simulink library "rov_design_analysis"  (Simulink 6.0)
settings: Solver=ode45  SolverMode=SingleTasking  StartTime=0.0  StopTime=10.0  RelTol=1e-3
undefined symbols (not defined in the file or in its folder): amp, At, B, Bt, Ct, cycles, D, den, DL, Do, DQ, DQL, freq, frtest, I, L, m, M, Ma, magnitude, MaU, Mt, nmiss, num, phase, rg, sigbuilder_block, slcm, T, W, xb, xg, Xudot, yb, yg, Yvdot, zb, zg, Zwdot
libraries: simulink_extras x32, simulink x27, rov_design_analysis x15, marine_gnc x10, dspmtrx2 x6, dspstat3 x4
(part 1 of 9)
Description:
  | jkgkh
settings Model: LastModifiedBy=c chin
settings OptimizationCC: BooleanDataType=off
settings DebuggingCC: SolverPrmCheckMsg=none
settings HardwareCC: TargetUnknown=on

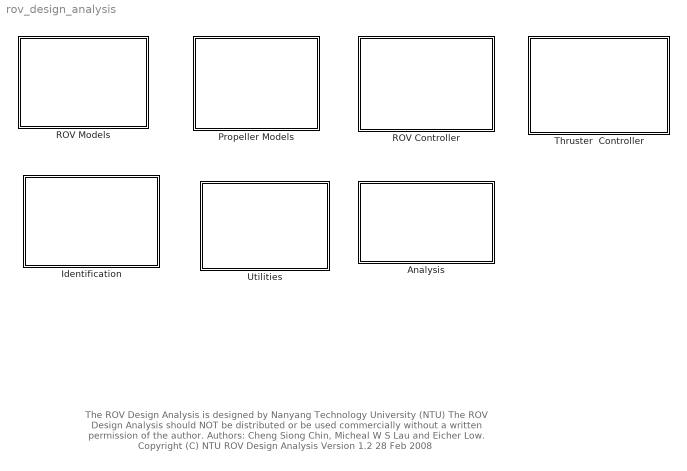
== system rov_design_analysis ==
  note: The ROV Design Analysis is designed by
      |
      |   Nanyang Technology University (NTU)
      |
      |
      | The ROV Design Analysis should NOT be distributed or be
      | used commercially without a written permission of the author.
      |
      |
      | Authors: Cheng Siong Chin, Micheal W S Lau
      | and  Eicher Low.
      |  Copyright (C)  NTU
      |
      |  ROV Design Analysis Version 1.2
      |  28 Feb 2008
  Analysis : Subsystem  AncestorBlock=rov_design_analysis/Scope
  Identification : Subsystem  AncestorBlock=rov_design_analysis/Scope
  Propeller Models : Subsystem  AncestorBlock="marine_gnc/Control/Dynamic  Positioning"
  ROV Models : Subsystem  AncestorBlock=marine_gnc/Control/Autopilots
  "ROV Controller " : Subsystem
  Thruster  Controller : Subsystem  AncestorBlock=|
      | rov_design_analysis/ROV Controller
      | Design
      | Applications
  Utilities : Subsystem  AncestorBlock=rov_design_analysis/ROV Modelling

== system rov_design_analysis/Analysis ==
  Linear/Nonlinear ROV Analysis : Subsystem  AncestorBlock=rov_design_analysis/Analysis/9. Design scaling
      settings: OpenFcn=|
      | clc
      | 
      | cd c:\Matlab7\toolbox\rov_design_analysis\gui
      | rov_property2
      mask Display: disp('ROV Property Analysis')
  Model Info : Subsystem  AncestorBlock=|  LoadFcn=slcm LoadBlock;  InitFcn=slcm('UpdateAllCMBlocksInThisModelInit')  mask(CMBlock){InitialSaveTempField=, InitialBlockCM=None, BlockCM=None, Frame=on, SaveTempField=, DisplayStringWithTags=|, MaskDisplayString=Reference:\n\nC. S. Chin, M. W. S. Lau, E. Low, G. G. Seet.\n Software for Modelling and Simulation of a Remotely Operated Vehicle, International Journal\nof Simulation Modelling, Vol.5, No. 3, p114-125, Sept 2006.\n\nAuthor: C.S.Chin\n27-Mar-2008 08:24:59, HorizontalTextAlignment=Left, LeftAlignmentValue=0.02, SourceBlockDiagram=rov_design_analysis, TagMaxNumber=20, CMTag1=, CMTag2=, CMTag3=, CMTag4=, CMTag5=, CMTag6=, CMTag7=, CMTag8=, CMTag9=, CMTag10=, CMTag11=, CMTag12=, CMTag13=, CMTag14=, CMTag15=, CMTag16=, CMTag17=, CMTag18=, CMTag19=, CMTag20=}
      | rov_design_analysis/ROV
      | Models/1. Nonlinear RRC ROV- unperturbed
      | (6DoF)/Model Info
      mask DisplayStringWithTags=|
      | Reference:\n
      | C. S. Chin, M. W. S. Lau, E. Low, G. G. Seet.\n Software for Modelling and Simulation of a Remotely Operated Vehicle, International Journal
      | of Simulation Modelling, Vol.5, No. 3, p114-125, Sept 2006.\n
      | %<Creator>Author: C.S.Chin
      | %<LastModificationDate>
      mask help: This block allows revision control information to be displayed within the model.
      settings: CopyFcn=slcm CopyBlock;  DeleteFcn=slcm Cancel;  PostSaveFcn=slcm('UpdateAllCMBlocksInThisModel')  NameChangeFcn=slcm Rename;  OpenFcn=slcm
      mask Display: text(str2num(LeftAlignmentValue), 0.5, MaskDisplayString, 'HorizontalAlignment', HorizontalTextAlignment)

== system rov_design_analysis/Identification ==
  Frequency Response Analysis : Subsystem
      mask Display: disp('Frequency Response \n Analysis')
  "Kalman filter  " : Subsystem  AncestorBlock=marine_gnc/Navigation/Observers/Kalman filter based autopilot wave filter  mask{lambda=0.1, w_o=1.0, T_b=1000, K=0.1, T=100, r=1, q1=100, q2=0.01, q3=0.01, P0=1*eye(5)}
      mask prompts: lambda "Relative damping ratio of wave spectrum: lambda"; w_o "Peak frequency of wave spectrum: w_o (rad/s)"; T_b "Bias time constant: T_b (s)"; K "Nomoto gain constant: K (1/s)"; T "Nomoto time constant: T (s)"; r "Compass variance: r"; q1 "Wave model variance: q1"; q2 "Ship model variance: q2"; q3 "Bias model variance: q3"; P0 "Initial covariance matrix"
      mask help:
      | Copyright (C) 2006 NTU
      | Author:  C.S.Chin
      mask Display: disp('Kalman filter')
  kalman filter- observer + i/o noise : Subsystem
      mask Display: disp('Kalman Filter')

== system rov_design_analysis/Propeller Models ==
  1.  propeller with motor characteristics - 1DoF (account for dynamic variation in ua,up) : Subsystem
      mask Type: Open-water propeller characteristics
      mask Description:
      | 1> Calculate the thrust and torque of a fixed pitch propeller, based on a polynomial representation of thrust and torque coefficients Kt and Kq from the open-water
      | characteristics. Kt and Kq are defined as polynomials alpha and beta in the advance number J=ua/(nD):
      | Kt =alpha(1)*J + alpha(2)
      | Kq =beta(1)*J + beta(2)
      | where n is the shaft speed, D the propeller diameter and ua the advance velocity of the propeller. The relationship between the thrust Ta and torque Qa are:
      | 
      | Ta = p*D^4*alpha(2)*n*|n| - p*D^3*alpha(1)*ua/(1+aT)
      | Qa = p*D^5*beta(2)*n*|n| - p*D^4*beta(1)*ua /(1+aQ)
      | where p is the density of water , n is the rotational speed of the propeller, aQ and aT are the constant used to account for dynamic variation in axial water speed.
      | 
      | 2> Calculate the Electrical DC Motor shaft equation:
      | Jdot*ndot+Km*Ke*n/Rm=Km*Vm/Rm-Qa
      | where Jm, Km, Ke, Rm are the motor constant and Vm is the voltage input.
      | 
      | 3>Calculate the axial flow velocity, up of the propeller
      | mt*updot-dto*up+dt|up|(up-ua)=Ta
      | where mt=gamma*p*Ap*l, gamma is an empirically determined added
      | mass coefficent, dt=2*p*Ap and advance velocity of propeller
      | 
      | ua=(1-W)u.
      | where W>0 is the wake fraction number (typical 0.1-0.4) and u is the ROV surge velocity.
      | 
      | *Note that ua is the advance velocity at the upstream of the propeller while up is axial
      |  velocity at the propeller. Details of the derivation can be found in:
      | 
      | [1] T.I.Fossen, M Blanke, Nonlinear output feedback control of underwater vehicle
      | propellers feedback form estimated axial flow velocity, IEEE Journal of Oceanic
      | Engineering, Vol 25, No.2, 2000.
      | 
      | Copyright (C) 2006 NTU, Author: C.S.Chin
      mask Display:
      | port_label('input', 1, 'volt [v]')
      | port_label('input', 2, 'vel [m/s & rad/s]')
      | port_label('output', 1, 'Ta [N]')
      | port_label('output', 2, 'Qa [Nm]')
      | port_label('output',3, 'ua[m/s]')
  2. propeller with motor characteristics - 1DoF (account for ua only) : Subsystem  AncestorBlock=|
      | rov_design_analysis/Propeller
      | Models/6. propeller with motor
      | characteristics
      | (account for ua)
      mask Type: Open-water propeller characteristics
      mask Description:
      | 1> Calculate the thrust and torque of a fixed pitch propeller, based on a polynomial representation of thrust and torque coefficients Kt and Kq from the open-water
      | characteristics. Kt and Kq for both thrust and torque are defined as:
      | 
      | Ktdo =p*Ap*l / (40*Kr) ,  Ktd=p*Ap/(800*Kr^2)         (Forward)
      | Ktdo = -p*Ap*l/(54Kr)  , Ktd=-p*Ap/(1458*Kr^2)       (Reverse)
      | 
      | Kqdo=p*Ap*l*D/(40*Kr) , Kqd=p*Ap*D/(800*Kr^2)     (Forward)
      | Kqdo=-p*Ap*l*D/(54*Kr), Kqd=-p*Ap*D/(1458*Kr^2)  (Reverse)
      | 
      | where p is the density of seawater=1024kg/m^3, l is the characteristic length =0.1m
      | Ap the propeller cross-sectional area, D is the propeller diameter =0.1m,
      | Kr=1.923, and  ua is the advance velocity of the propeller.
      | 
      | ua=(1-W)u
      | 
      | where W> 0 (=0.4) is the wake fraction number and u is the ROV surge velocity.
      | 
      | The relationship between the thrust Ta and torque Qa are:
      | 
      | Ta= Ktdo * ndot+Ktd*n|n|
      | Qa =Kqdo*ndot+Kqt*n|n|
      | where  n is the rotational speed of the propeller,
      | Ktdo=0.0104 ,Ktd=0.0027, Kqdo=0.00104, Kqd=0.00149.
      | 
      | 2> Calculate the Electrical DC Motor shaft equation:
      | Jdot*ndot+Kv*n=Km*Vm/Rm-Qa
      | where Jm = shaft inertia,
      |             Rm = motor resistance,
      |              Kv  = viscous friction coefficient,
      |             Vm = voltage input
      |             Qa =  torque output.
      | 
      | Copyright (C) 2006 NTU, Author: C.S.Chin
      mask Display:
      | port_label('input', 1, 'volt [v]')
      | port_label('input', 2, 'vel [m/s & rad/s]')
      | port_label('output', 1, 'Ta [N]')
      | port_label('output', 2, 'Qa [Nm]')
      | port_label('output',3, 'ua[m/s]')
  3. propeller with motor characteristics - 1DoF (no account for ua,up) : Subsystem
      mask Type: Propeller dynamic without considering axial velocity
      mask Description:
      | 1> Voltage input to motor:
      | 
      | Vm=Rm*I+Ke*Ohm+Lm*dI/dt
      | 
      | where Rm= motor resistance in Ohms
      |              Ke = motor  back emf constant in Vs/rad
      |              Lm= motor inductance in H
      |              I = motor current in A
      | 
      |  2> Propeller thrust (T) and torque (Q) output
      | 
      | T=Ktd*n|n|+Ktdo*n
      | Q=Kqd*n|n|+Kqdo*n
      | 
      | where n= rotational speed in rad/s
      | 
      | Copyright (C) 2006 NTU
      | Author:  C.S.Chin
  4. Open-water propeller characteristics : Subsystem  AncestorBlock=marine_gnc/Models/Propulsion/Open-water propeller characteristics  mask(Open-water propeller characteristics){Par_Thruster_D=1, Par_Thruster_Ktp=[-0.1060 -0.3246 0.4594], Par_Thruster_Kqp=[-0.0186 -0.0399 0.0680], Par_Thruster_reverse_reduction=0.8, Glob_rhow=1025}
      mask prompts: Par_Thruster_D "Thruster diameter [m]"; Par_Thruster_Ktp "Kt polynomial Ktp"; Par_Thruster_Kqp "Kq polynomial Kqp"; Par_Thruster_reverse_reduction "Reverse direction thrust reduction factor [-]"; Glob_rhow "Density of seawater [kg/m^3]"
      mask help:
      | Calculate the thrust and torque of a fixed pitch propeller, based on a polynomial representation of thrust and torque coefficients Kt and Kq from the open-water characteristics. Kt and Kq are defined as polynomials Ktp and Kqp in the advance number J=Va/(nD):
      |
      | Kt = Ktp(1)*J^2 + Kqp(2)*J + Kqp(3)
      | Kq = Kqp(1)*J^2 + Kqp(2)*J + Kqp(3)
      |
      | where n is the shaft speed, D the propelelr diameter and Va the advance velocity of the propeller. The relationship between the thrust T and torque Q and the coefficients Kt and Kq is:
      |
      | T = Kt*rho*D^4
      | Q = Kq*rho*D^5
      |
      | where rho is the density of water. See help for details.
      |
      | Copyright (C) 2005 NTNU
      |
      | Author: Oyvind Notland Smogeli
      mask Help:
      | <p>
      | <b>Part of the Marine Systems Simulator: MSS</b></p>
      | <p>Calculate the thrust and torque of a fixed pitch propeller, based on a polynomial
      | representation of thrust and torque coefficients from the open-water
      | characteristics.</p>
      | <p><b>Inputs: </b> </p>
      | <p>n: [1/s] Propeller shaft speed<br>
      | Va: [m/s] Propeller advance speed</p>
      | <p><b>Outputs: </b> </p>
      | <p>T: [N] Propeller thrust<br>
      | Q: [Nm] Propeller torque<p><b>Model validity:</b><p>The model gives the thrust and torque from a polynomial of the form:<p>T = sign(n)*[T_nn*n^2 + T_Vn*Va*n + T_VV*Va^2]<br>Q = sign(n)*[Q_nn*n^2 + Q_Vn*Va*n + Q_VV*Va^2]<p>If the expression in brackets becomes negative, it is set to zero.
      | Propeller windmilling is therefore not accounted for.
      | The thrust is modified by a reduction factor when the thruster is
      | reversed (n &lt; 0), and the torque kept unmodified. Negative advance velocities
      | are treated as zero.<p>The coefficients are:<p>T_nn = Ktp(3)*rhow*D^4<br>T_Vn = Ktp(2)*rhow*D^3<br>T_VV = Ktp(1)*rhow*D^2<br>Q_nn = Kqp(3)*rhow*D^5<br>Q_Vn = Kqp(2)*rhow*D^4<br>Q_VV = Kqp(1)*rhow*D^3<p>
      | where rhow is the density of seawater, D the propeller diameter, and
      | Ktp and Kqp are the polynomials defined in the mask:<p>Kt = Ktp(1)*J^2 + Kqp(2)*J + Kqp(3)<br>Kq = Kqp(1)*J^2 + Kqp(2)*J + Kqp(3)<p>where J is the advance number, J = Va/(n*D).
      | The relationship between the thrust and torque and the coefficients Kt and Kq
      | is:<p>T = Kt*rhow*D^4<br>Q = Kq*rhow*D^5<p>Example input data for a
      | Wageningen B-series propeller with pitch ratio P/D = 1, number of blades Z = 4 and
      | expanded blade area ratio EAR = 0.7:<p>Ktp = [-0.1060 -0.3246 0.4594]<br>Kqp = [-0.0186 -0.0399 0.0680]<br>
      | reverse_reduction = 0.8<p>
      | <b>Copyright NTNU 2005</b></p>
      | <p><b>Author:</b> Oyvind N. Smogeli, 2005-05-03</p>
      mask Display:
      | image(imread('propeller.jpg'))
      | port_label('input', 1, 'n [1/s]')
      | port_label('input', 2, 'Va [m/s]')
      | port_label('output', 1, 'T [N]')
      | port_label('output', 2, 'Q [Nm]')
  5. first-order thruster dynamic - 4 DoF : Subsystem  AncestorBlock=|
      | rov_design_analysis/ROV Controller
      | Design
      | Applications/2. Passivity-based 
      | and 
      | sliding mode control/Subsystem2
      mask Type: First-Order Dynamic Thruster Model
      mask Description:
      | Thruster transfer function,
      | 
      | GT= 0.97/(0.02s+1)
      | 
      | Copyright (C) 2006 NTU
      | Author:  C.S.Chin
  6. first order motor dynamic- 1DoF (no account for ua,up) : Subsystem  AncestorBlock=|
      | rov_design_analysis/Controller
      | Design
      | Applications/shaft speed control/Speed control
      mask Type: Thruster modeling
      mask Description:
      | 1> First-order motor model:
      | 
      | Qmdot=1/Tm*(Qc-Qm)
      | 
      | where  Tm = time constant in s
      |               Qc = desired torque in Nm
      |               Qm = motor torque in Nm
      | 
      | 2> Rotational dynamic with friction
      | 
      | Jm*ndot=Qm-Q-Ke*n
      | 
      | where Jm= motor shaft inertia in Nms^2/rad
      |              Qm=motor torque in Nm
      |              Q= propeller load torque in Nm
      |              Ke=  motor back emf constant in Vs/rad
      | 
      | 3> Propeller load torque
      | 
      | Q=p*D^5*Kqd*n|n|
      | 
      | where p=seawater density in kg/m^3
      |             D=propeller diameter in m
      |             n=rotational speed in rad/s
      |             Kqd=torque constant
      | 
      | 4> Propeller thrust
      | 
      | T=p*D^4*Ktd*n*|n|
      | 
      | where p=seawater density in kg/m^3
      |             D=propeller diameter in m
      |             n=rotational speed in rad/s
      |             Ktd=thrust constant
      | 
      | Reference:
      | [1] O. Smogeli & A. J. Sorensen, Presentation note on Propulsion control, NTNU.
      | 
      | Copyright (C) 2006 NTU
      | Author:  C.S.Chin
  parameters Info : simulink/Model-Wide Utilities/Model Info  InitialBlockCM=None  BlockCM=None  Frame=on  DisplayStringWithTags=|  HorizontalTextAlignment=Left  LeftAlignmentValue=0.02  SourceBlockDiagram=rov_design_analysis  TagMaxNumber=20
      | Parameters used for RRC ROV2 Propeller
      | 1>p=1024 kg/m^3
      | 2>l=0.01m
      | 3>D=0.1m
      | 4>Kr=2.14
      | 5>W=0.4
      | 6> Ktdo=0.00094, Ktd=0.0022, Kqdo=0.000094, Kqd=0.00022
      | 7>Km=12.562 Nm/A (forward), 8.759 Nm/A (reverse)
      | 8>Jm=0.0492 Nms^2/rad (forward), 0.0492 Nms^2/rad (reverse)
      | 9>Rm=2.4 Ohms (forward) 2.4 Ohms(reverse)
      | 10>Kv=1.6 Nms/rad (forward) 0.978 Nms/rad (reverse)\n
      | Copyright (C) 2006 NTU
      | Author:  C.S.Chin
      | %<LastModificationDate>
  solver Info : simulink/Model-Wide Utilities/Model Info  InitialBlockCM=None  BlockCM=None  Frame=on  DisplayStringWithTags=|  HorizontalTextAlignment=Center  LeftAlignmentValue=0.5  SourceBlockDiagram=rov_design_analysis  TagMaxNumber=20
      | For all propeller simulation: \n
      | Use solver: ode23(Bogacki-Shampine)
      | Relative tolerance: 1e-8

== system rov_design_analysis/ROV Models ==
  " Linear RRC ROV- unperturbed (6DoF)" : Subsystem  AncestorBlock=rov_design_analysis/ROV Models/1. Six DOF RRC ROV- unperturbed
      mask Display:
      | disp('ROV')
      | image(imread('/rov_design_analysis/fig/ROVRRC2.jpg'));
      | color('black');port_label('input',1,'thrust')
      | color('black');port_label('input',2,'pos')
      | color('black');port_label('output',1,'vel')
  " Pseudo Inverse (n X n-j), j<n" : Subsystem  mask(Insert Pseudo Inverse Matrix (for non-square system)){invT=0}
      mask prompts: invT "Insert matrix"
      mask help:
      | Calculate pseudo inverse of  T with dimensions n x (n-j) where j<n.
      |
      | invT=pinv(T)
      |
      | Copyright (C) 2006 NTU
      | Author:  C.S.Chin
      mask Display:
      | disp('Thrust Optim \n (Pseudo-Inverse)')
      | color('black');port_label('input',1,'volt-(n-j)')
      | color('black');port_label('output',1,'volt-(n)')
  " ROMEO ROV (6DoF)   " : Subsystem
      mask Display:
      | disp('ROMEO ROV')
      | image(imread('/rov_design_analysis/fig/ROMEO.jpg'))
      | color('white');port_label('input',1,'ubar_i')
      | color('white');port_label('input',2,'thrust')
      | color('white');port_label('input',3,'MCD_select')
      | color('white');port_label('input',4,'eout')
      | color('white');port_label('input',5,'bout_p')
      | 
      | color('white');port_label('output',1,'vel')
      | color('white');port_label('output',2,'boutdot')
  1. Nonlinear RRC ROV- unperturbed (6DoF) : Subsystem  AncestorBlock=rov_design_analysis/ROV Modelling/Heading autopilot/linear system1
      mask Display:
      | disp('ROV')
      | image(imread('/rov_design_analysis/fig/ROVRRC2.jpg'));
      | color('black');port_label('input',1,'thrust')
      | color('black');port_label('input',2,'pos')
      | color('black');port_label('output',1,'vel')
  3. Compute tether force : Subsystem
      settings: OpenFcn=|
      | clc
      | cd c:\Matlab7\toolbox\rov_design_analysis\\gui;
      | 
      | forceCal
      mask Display: disp('double-click \n to compute \n tether force (RRC ROV)')
  4.  Thruster Configuration Matrix (n X n) : Subsystem  mask(Thruster Configuration Matrix ){T=}
      mask prompts: T "Insert Thruster Configuration Matrix"
      mask help:
      | Provide the thruster configuration matrix using summation of forces and moment about the vehicle's C.G.
      |
      | Copyright (C) 2006 NTU
      | Author:  C.S.Chin
      mask Display:
      | disp('Thruster \n Configuration')
      | 
      | color('black');port_label('input',1,'volt-in')
      | color('black');port_label('output',1,'volt-out')
  5. First -order current velocities : Subsystem  mask{attackA=0, waveA=0}
      mask prompts: attackA "Angle of Attack"; waveA "Wave direction"
      mask help:
      | Provide the first-order cuurent input in x,y,z, yaw DoFs.
      |
      | Copyright (C) 2006 NTU
      | Author:  C.S.Chin
  "JHU ROV (6DoF)   " : Subsystem
      mask Display:
      | disp('JHU ROV')
      | image(imread('/rov_design_analysis/fig/JHUROV.jpg'))
      | color('white');port_label('input',1,'ubar_i')
      | color('white');port_label('input',2,'thrust')
      | color('white');port_label('input',3,'MCD_select')
      | color('white');port_label('input',4,'eout')
      | color('white');port_label('input',5,'bout_p')
      | 
      | color('white');port_label('output',1,'vel')
      | color('white');port_label('output',2,'boutdot')
  "Nonlinear RRC ROV - Perturbed (6DoF)   " : Subsystem
      mask Display:
      | disp('ROV')
      | image(imread('/rov_design_analysis/fig/ROVRRC2.jpg'));
      | color('white');port_label('input',1,'ubar_i')
      | color('white');port_label('input',2,'thrust')
      | color('white');port_label('input',3,'MCD_select')
      | color('white');port_label('input',4,'eout')
      | color('white');port_label('input',5,'bout_p')
      | 
      | color('white');port_label('output',1,'vel')
      | color('white');port_label('output',2,'boutdot')
  Sine perturbation-1DoF : Subsystem  AncestorBlock=rov_design_analysis/ROV Models/6. First -order current velocities
  Thruster Configuration Matrix of RRC ROV  (6X4) : Subsystem  AncestorBlock=|
      | rov_design_analysis/Thruster
      | Modelling/Thruster Configuration Matrix
      | (6X4)
      mask Display:
      | disp('Thruster \n (ROV)')
      | 
      | color('black');port_label('input',1,'beta')
      | color('black');port_label('input',2,'delta')
      | color('black');port_label('input',3,'gamma')
      | color('black');port_label('input',4,'epsilon')
      | color('black');port_label('input',5,'alpha')
      | 
      | color('black');port_label('output',1,'T(.)')

== system rov_design_analysis/ROV Controller  ==
  " Hamiltonian  Interconnection-Damping Assignment  - 2 DoF" : Subsystem  mask{A=}
      mask prompts: A "Needed to invoke OpenFcn from the browser:"
      settings: OpenFcn=|
      | cd c:\matlab7\toolbox\rov_design_analysis\controller
      | open IDA
      mask Display: disp('Hamiltonian- IDA')
  " Multi-controller selection -  4 DoF" : Subsystem  Description=f(x)
  " Open-loop ROV - 6 DoF" : Subsystem  AncestorBlock=|  mask{A=}
      | rov_design_analysis/ROV Controller
      | / PID control 
      | on semi-submersible
      mask prompts: A "Needed to invoke OpenFcn from the browser:"
      settings: OpenFcn=|
      | cd c:\matlab7\toolbox\rov_design_analysis\vechicle_model
      | open rov_openloop
      mask Display: disp('Open-Loop \n ROV \n System ');
  Adaptive PD  Cascaded  Controller - 6 DoF : Subsystem  AncestorBlock=|
      | rov_design_analysis/ROV Controller
      | /P-Decoupled Single
      | Controller
      settings: OpenFcn=|
      | cd c:\matlab7\toolbox\rov_design_analysis\controller
      | open Adaptive_cascade_rov
      mask Display: disp('Adaptive \n Cascaded \n controller')
  Hybrid Control- one DoF : Subsystem  AncestorBlock=|
      | rov_design_analysis/ROV Controller
      | /Nonlinear-Sliding-Mode
      | Cascaded 
      | Controller
      settings: OpenFcn=|
      | cd c:\matlab7\toolbox\rov_design_analysis\controller
      | open hybrid_cont
      mask Display: disp('Hybrid \n Controller')
  Nonlinear-Based PD  Cascaded  Controller - 6 DoF : Subsystem  AncestorBlock=|
      | rov_design_analysis/ROV Controller
      | /Adaptive PD Cascaded 
      | Controller
      settings: OpenFcn=|
      | cd c:\matlab7\toolbox\rov_design_analysis\controller
      | open MBNLC_cascade_rov
      mask Display: disp('Nonlinear Model-Based \n Cascaded \n controller')
  Nonlinear-Sliding-Mode Cascaded  Controller - 6 DoF : Subsystem  AncestorBlock=|
      | rov_design_analysis/ROV Controller
      | /Nonlinear-Based PD 
      | Cascaded 
      | Controller
      settings: OpenFcn=|
      | cd c:\matlab7\toolbox\rov_design_analysis\controller
      | open Slidingmode_cascade_rov
      mask Display: disp('Nonlinear Sliding-Mode \n Cascaded \n controller')
  P-Decoupled  Cascaded loop Controller  - 6 DoF : Subsystem
      settings: OpenFcn=|
      | cd c:\matlab7\toolbox\rov_design_analysis\controller
      | open P_decouple_cascade_rov
      mask Display: disp('P-Decoupled \n Cascaded \n controller')
  "P-Decoupled  Single loop Controller - 6 DoF " : Subsystem  AncestorBlock=|
      | rov_design_analysis/ROV Controller
      | /P-Decoupled Cascaded
      | Controller
      settings: OpenFcn=|
      | cd c:\matlab7\toolbox\rov_design_analysis\controller
      | open P_decouple_single_rov
      mask Display: disp('P-Decoupled \n Single \n controller')
  PID  -  4 DoF : Subsystem  AncestorBlock=|
      | rov_design_analysis/ROV Controller
      | Design
      | Applications/1. Heading autopilot/controller/PD for all
  PID  - 6 DoF : Subsystem  AncestorBlock=rov_design_analysis/ROV Controller /PID x 4
  ROV design  in earth fixed frame  PID - 6 DoF : Subsystem  AncestorBlock=rov_design_analysis/ROV Controller / Open-loop ROV  mask{A=}
      mask prompts: A "Needed to invoke OpenFcn from the browser:"
      settings: OpenFcn=|
      | cd c:\matlab7\toolbox\rov_design_analysis\controller
      | open PID_earth_NCD
      mask Display: disp('ROV-Earth Fixed \n PID Control ');

== system rov_design_analysis/Thruster  Controller ==
  1. Propeller thrust control - one DoF : Subsystem
      settings: OpenFcn=|
      | cd c:\matlab7\toolbox\rov_design_analysis\controller
      | open thruster_controller
      mask Display: disp('Propeller Thrust Control')
  2. Thruster Allocation- RRC ROV : Subsystem
      mask Display: disp('Thruster Allocation')

== system rov_design_analysis/Utilities ==
  6 DoF comparison : Subsystem  AncestorBlock=marine_gnc/Utilities/Simulation tools/6DOF comparison
      mask Type: 6DOF comparison
      mask Description:
      | Compare two 6DOF signals (i.e. motion or force). To view the signals, open the scope inside the block.
      | 
      | Copyright (C) 2006 NTU
      | Author:  C.S.Chin
  6 to 4 DoF : Subsystem
  6 to 4 or 2 DoF : Subsystem
  "Body Velocity Scope (6 DoF)  " : Subsystem  AncestorBlock=|
      | rov_design_analysis/Controller
      | Design/Heading autopilot/Outcome
      | Velocity
      | Scope1
      mask Display: disp('Body\nVelocity\nScope')
  "Earth Position  Scope (6 DoF) " : Subsystem  AncestorBlock=|
      | rov_design_analysis/ROV Controller
      | Design
      | Applications/4. Lyapunov PID/Outcome
      | Velocity
      | Scope1
      mask Display: disp('Earth\nPosition\nScope')
  "Euler Transformation 4 DoF  " : Subsystem  AncestorBlock=rov_design_analysis/Scope Utilities/Euler Transformation
  Euler Transformation 6 DoF : Subsystem  AncestorBlock=|
      | rov_design_analysis/Controller
      | Design/Heading autopilot/Body-fixed to
      | Earth_fixed
      | Transformation1
  Inverse Euler Transformation 4 DoF : Subsystem
  Joystrick (4 DoF) : Subsystem
  Modes indicator-hort/vert/station - 6 DoF : Subsystem  Description=f(x)
  Process Capability  (1 DoF) : Subsystem  AncestorBlock=|
      | rov_design_analysis/Scope
      | Utilities/Z-score (1 DOF)
  Switching sequence : Subsystem
      mask Display: disp('Dwell \n Sequence')
  Switching sequence - Controller : Subsystem  mask{t1=0, t2=0, t3=0, t4=0, t5=0}
      mask help:
      | Switching  at each time instant ( t1 to t5).
      | Maximum 5 controllers (labeled as 1,2,3,4,5).
      mask Display: disp('Switching \n Sequence')
  Time capture : Subsystem  mask{t=<empty>}
      mask prompts: t "Time in seconds"
      mask help:
      | Output time in seconds to variable ' t '
      |
      | Copyright (C) 2006 NTU
      | Author:  C.S.Chin
      mask Display: disp('Time \n capture')
  Unit Conversion : Subsystem  AncestorBlock=marine_gnc/Utilities/Math Operations/Unit Conversion  mask(Unit Conversion){in=<empty>}
      mask prompts: in "Convert"
      mask help:
      | Block to convert units. If the input in is a vector,
      | all the components are converted using the same conversion factor.
      |
      | Copyright (C) 2006 NTU
      | Author:  C.S.Chin
      mask init:
      | if  in==1,
      | k=pi/180;
      | elseif  in==2,
      | k=180/pi;
      | elseif in==3,
      | k = .5145;
      | elseif in ==4,
      | k = 1/.5145;
      | elseif in==5,
      | k=9.81
      | end
      mask StyleString: popup(<empty>)
  Z-score (1 DoF) : Subsystem
  pipe tracking profile  (4 DoF) : Subsystem  AncestorBlock=rov_design_analysis/Scope/pipe tracking profile
      mask Display: disp('Pipeline Tracking \n (manual)')
  pipe tracking profile  (6 DoF) : Subsystem  AncestorBlock=|
      | rov_design_analysis/Scope
      | Utilities/pipe tracking
      | profile 
      | (4 inputs)
      mask Display: disp('Pipeline Tracking \n (manual)')
  "pipeline  tracking planner  (6 DoF) " : Subsystem  AncestorBlock=|
      | rov_design_analysis/ROV Controller
      | Design
      | Applications/1. Heading autopilot/pipe tracking
      | profile
      | (Auto)
      mask Display: disp('Pipeline \n Planner')

== system rov_design_analysis/Analysis/Linear/Nonlinear ROV Analysis ==

== system rov_design_analysis/Analysis/Model Info ==
  EmptySubsystem : Subsystem

== system rov_design_analysis/Identification/Frequency Response Analysis ==
  1.open : Subsystem  AncestorBlock=rov_design_analysis/Identification/Frequency Response Analysis/load example
      settings: OpenFcn=|
      | nmiss=0;
      | cycles=1;
      | frtest=10;
      | cd c:\matlab7\toolbox\rov_design_analysis\FRA
      | open freq_thruster
      mask Display: disp('Open \n "freq_thruster.mdl" ')
  2.Plot Bode : Subsystem  AncestorBlock=rov_design_analysis/sensor/Frequency Response Analysis/output ss model
      settings: OpenFcn=|
      | cd c:\Matlab7\toolbox\rov_design_analysis\m_file;
      | 
      | run bode_fit_thruster
      mask Display: disp('Plot Bode')
  3. Plot Mag : Subsystem  AncestorBlock=rov_design_analysis/Identification/Frequency Response Analysis/More Info
      settings: OpenFcn=|
      | cd c:\Matlab7\toolbox\rov_design_analysis\FRA
      | figure
      | run make25;
      mask Display: disp('Plot mag at frtest=10rad/s')
  Correlation Frquency Analyzer : Subsystem
  Model Info1 : Subsystem  LoadFcn=slcm LoadBlock;  InitFcn=slcm('UpdateAllCMBlocksInThisModelInit')  mask(CMBlock){InitialSaveTempField=, InitialBlockCM=None, BlockCM=None, Frame=on, SaveTempField=, DisplayStringWithTags=|, MaskDisplayString=Frequency Response Analysis \n\nFrequency response analysis is the technique whereby a sinusoidal test signal is used\nto  measure points on the frequency response of a  transfer function or \nimpedance function. \n\nThe basic set-up in which a sine wave u(t) is applied to a system with transfer \nfunction G(s).After the transients due to initial conditions have decayed  away,\n the output y(t) becomes a sine wave but with a different magnitude \nY and a relative phase. \n\nThe magnitude and phase of the output y(t) are in fact related to the transfer function G(s) \nat the frequency w rad/s of the input sinusoid.\n\nStep:\n1> Insert a new model for simulation. \nClick the "freq_thruster.mdl" and inset new model in the "system under test" . \n Then click "start simulation" \n\n2>Double-click "Plot Bode". \n\n3> Double-click "Plot mag at frtest" (e.g. frtest=10 rad/s)  \n\nCopyright (C) 2006 NTU\nAuthor:  C.S.Chin\n27-Mar-2008 08:24:59, HorizontalTextAlignment=Left, LeftAlignmentValue=0.02, SourceBlockDiagram=rov_design_analysis, TagMaxNumber=20, CMTag1=, CMTag2=, CMTag3=, CMTag4=, CMTag5=, CMTag6=, CMTag7=, CMTag8=, CMTag9=, CMTag10=, CMTag11=, CMTag12=, CMTag13=, CMTag14=, CMTag15=, CMTag16=, CMTag17=, CMTag18=, CMTag19=, CMTag20=}
      mask DisplayStringWithTags=|
      | Frequency Response Analysis \n
      | Frequency response analysis is the technique whereby a sinusoidal test signal is used
      | to  measure points on the frequency response of a  transfer function or
      | impedance function. \n
      | The basic set-up in which a sine wave u(t) is applied to a system with transfer
      | function G(s).After the transients due to initial conditions have decayed  away,
      |  the output y(t) becomes a sine wave but with a different magnitude
      | Y and a relative phase. \n
      | The magnitude and phase of the output y(t) are in fact related to the transfer function G(s)
      | at the frequency w rad/s of the input sinusoid.\n
      | Step:
      | 1> Insert a new model for simulation.
      | Click the "freq_thruster.mdl" and inset new model in the "system under test" . \n Then click "start simulation" \n
      | 2>Double-click "Plot Bode". \n
      | 3> Double-click "Plot mag at frtest" (e.g. frtest=10 rad/s)  \n
      | Copyright (C) 2006 NTU
      | Author:  C.S.Chin
      | %<LastModificationDate>
      mask help: This block allows revision control information to be displayed within the model.
      settings: CopyFcn=slcm CopyBlock;  DeleteFcn=slcm Cancel;  PostSaveFcn=slcm('UpdateAllCMBlocksInThisModel')  NameChangeFcn=slcm Rename;  OpenFcn=slcm
      mask Display: text(str2num(LeftAlignmentValue), 0.5, MaskDisplayString, 'HorizontalAlignment', HorizontalTextAlignment)
  Sine Wave : Sin  Frequency=frtest  SampleTime=0
  System under test : Subsystem
      mask Display: image(imread('propeller.jpg'))
  mag : ToWorkspace  VariableName=mag  SampleTime=-1  SaveFormat=Array
  phase : ToWorkspace  VariableName=phase  SampleTime=-1  SaveFormat=Array
  wires:
  Correlation Frquency Analyzer/2(deg) -> phase/1
  Correlation Frquency Analyzer/1(mag) -> mag/1
  Sine Wave/1 -> Correlation Frquency Analyzer/1(Sine wave), System under test/1(In1)
  System under test/1(Out1) -> Correlation Frquency Analyzer/2(in)

== system rov_design_analysis/Identification/Kalman filter   ==
  note: compass transfer func
  sensor  input : Inport  Orientation=down  Port=1  LatchInput=off
  actual sens  input : Inport  Orientation=down  Port=2  LatchInput=off
  "  " : Math  Operator=transpose  SaturateOnIntegerOverflow=on
  "    " : Gain  Gain=1/r  SaturateOnIntegerOverflow=on
  "     " : Gain  Gain=1/r  SaturateOnIntegerOverflow=on
  0.5*(P+P') : Subsystem
  AP : Product  Multiplication=Matrix(*)  SaturateOnIntegerOverflow=on
  H' : Constant  Value=[0 1 1 0 0]
  H'*H : Product  Multiplication=Matrix(*)  SaturateOnIntegerOverflow=on
  Integrator5 : Integrator  InitialCondition=P0
  P*H' : Product  Inputs=**  Multiplication=Matrix(*)  SaturateOnIntegerOverflow=on
  P*H'*(1/r)*H*P : Product  Inputs=***  Multiplication=Matrix(*)  SaturateOnIntegerOverflow=on
  Product : Product  SaturateOnIntegerOverflow=on
  Sum : Sum  Inputs=|++  SaturateOnIntegerOverflow=on
  Sum10 : Sum  Inputs=|-+  SaturateOnIntegerOverflow=on
  Sum11 : Sum  Orientation=up  Inputs=|++  SaturateOnIntegerOverflow=on
  Sum2 : Sum  Orientation=left  Inputs=+|-  SaturateOnIntegerOverflow=on  InputSameDT=on
  Transpose : Math  Operator=transpose  SaturateOnIntegerOverflow=on
  "[-inf inf] to [-pi pi]" : marine_gnc/Utilities/Math Operations/[-inf inf] to [-pi pi]  Orientation=left
  matrices : Subsystem
  y_hat : Outport
  wires:
  matrices/1(A) -> AP/1
  "  "/1 -> H'*H/2  "H"
  "    "/1 -> P*H'*(1/r)*H*P/2
  P*H'/1 -> "     "/1
  H'*H/1 -> "    "/1
  H'/1 -> P*H'/2, H'*H/1, "  "/1  "H'"
  Sum2/1 -> "[-inf inf] to [-pi pi]"/1
  sensor  input/1 -> Sum2/1
  AP/1 -> Sum/1, Transpose/1
  Sum10/1 -> Integrator5/1
  Transpose/1 -> Sum/2  "PA'"
  Sum11/1 -> Sum10/2
  "     "/1 -> Product/1  "P*H'*inv(r)"
  matrices/2(EQE') -> Sum11/2
  Sum/1 -> Sum11/1
  "[-inf inf] to [-pi pi]"/1 -> Product/2
  Product/1 -> y_hat/1  "K*eps"
  P*H'*(1/r)*H*P/1 -> Sum10/1
  Integrator5/1 -> 0.5*(P+P')/1(P)  "P"
  0.5*(P+P')/1(P=P') -> AP/2, P*H'/1, P*H'*(1/r)*H*P/3, P*H'*(1/r)*H*P/1
  actual sens  input/1 -> Sum2/2

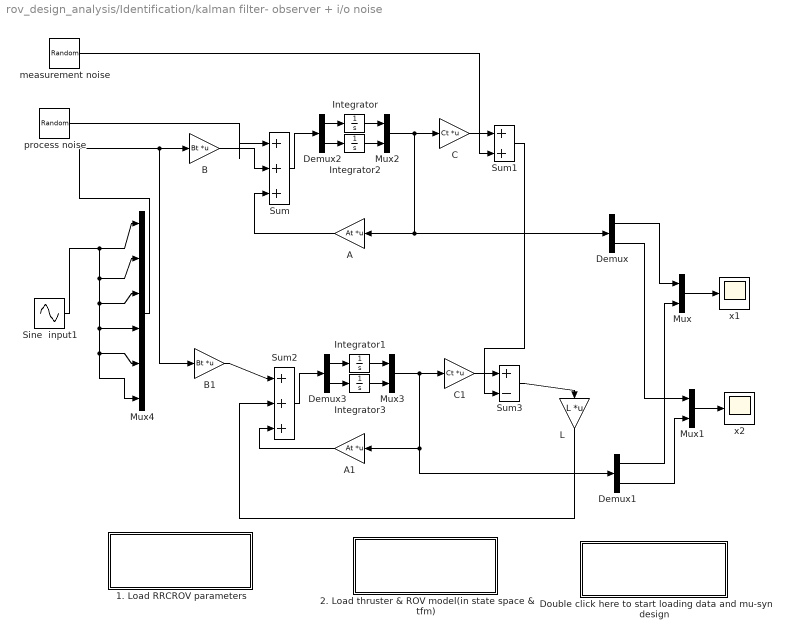
== system rov_design_analysis/Identification/kalman filter- observer + i/o noise ==
  1. Load RRCROV parameters : Subsystem  AncestorBlock=rov_design_analysis/Analysis/1. Load RRCROV2 parameters
      settings: OpenFcn=|
      | clc
      | cd c:\Matlab7\toolbox\rov_design_analysis\\mat_file ;
      | load rrcrovf;
      mask Display: disp('Load the\n RRCROV\n parameters')
  2. Load thruster & ROV model(in state space & tfm) : Subsystem  AncestorBlock=rov_design_analysis/Analysis/2. Load thruster & ROV model(in state space & tfm)
      settings: OpenFcn=|
      | cd c:\Matlab7\toolbox\rov_design_analysis\\m_file ;
      | run Analy_ss;
      mask Display: disp('Load Thruster & ROV \n (in ss & tfm) ')
  A : Gain  Orientation=left  Gain=At  Multiplication=Matrix(K*u)  SaturateOnIntegerOverflow=on
  A1 : Gain  Orientation=left  Gain=At  Multiplication=Matrix(K*u)  SaturateOnIntegerOverflow=on
  B : Gain  Gain=Bt  Multiplication=Matrix(K*u)  SaturateOnIntegerOverflow=on
  B1 : Gain  Gain=Bt  Multiplication=Matrix(K*u)  SaturateOnIntegerOverflow=on
  C : Gain  Gain=Ct  Multiplication=Matrix(K*u)  SaturateOnIntegerOverflow=on
  C1 : Gain  Gain=Ct  Multiplication=Matrix(K*u)  SaturateOnIntegerOverflow=on
  Demux{,1..3} (4 alike) : Demux  Outputs=2
  Double click here to start loading data and mu-syn design : Subsystem
      settings: OpenFcn=|
      | cd c:\matlab7\toolbox\rov_design_analysis\m_file;
      |  run kalman_data ;
      mask Display: disp('Load\nSystem data \n and \n determine kalman gain ')
  Integrator : Integrator  InitialCondition=0.5
  Integrator1 : Integrator  InitialCondition=0.5
  Integrator2 : Integrator  InitialCondition=-0.5
  Integrator3 : Integrator  InitialCondition=-0.5
  L : Gain  Orientation=down  Gain=L  Multiplication=Matrix(K*u)  SaturateOnIntegerOverflow=on
  Mux{,1..3} (4 alike) : Mux  Inputs=2
  Mux4 : Mux  Inputs=6
  Sine  input1 : Sin  SampleTime=0
  Sum : Sum  Inputs=|+++  SaturateOnIntegerOverflow=on  InputSameDT=on
  Sum1 : Sum  Inputs=|++  SaturateOnIntegerOverflow=on  InputSameDT=on
  Sum2 : Sum  Inputs=|+++  SaturateOnIntegerOverflow=on  InputSameDT=on
  Sum3 : Sum  Inputs=|+-  SaturateOnIntegerOverflow=on  InputSameDT=on
  measurement noise : RandomNumber  Variance=0.25  SampleTime=0
  process noise : RandomNumber  Variance=0.09  SampleTime=0
  x1 : Scope
  x2 : Scope
  wires:
  B/1 -> Sum/2
  A/1 -> Sum/3
  C/1 -> Sum1/2
  C1/1 -> Sum3/2
  B1/1 -> Sum2/1
  A1/1 -> Sum2/3
  L/1 -> Sum2/2
  Sum1/1 -> Sum3/1
  Sum3/1 -> L/1
  Demux/1 -> Mux/1
  Demux1/1 -> Mux/2
  Mux/1 -> x1/1
  Demux/2 -> Mux1/1
  Demux1/2 -> Mux1/2
  Mux1/1 -> x2/1
  process noise/1 -> Sum/1
  measurement noise/1 -> Sum1/1
  Demux2/1 -> Integrator/1
  Integrator/1 -> Mux2/1
  Demux2/2 -> Integrator2/1
  Integrator2/1 -> Mux2/2
  Sum/1 -> Demux2/1
  Mux2/1 -> C/1, A/1, Demux/1
  Demux3/1 -> Integrator1/1
  Integrator1/1 -> Mux3/1
  Demux3/2 -> Integrator3/1
  Integrator3/1 -> Mux3/2
  Sum2/1 -> Demux3/1
  Mux3/1 -> C1/1, A1/1, Demux1/1
  Mux4/1 -> B/1, B1/1
  Sine  input1/1 -> Mux4/1, Mux4/2, Mux4/3, Mux4/4, Mux4/5, Mux4/6

== system rov_design_analysis/Propeller Models/1.  propeller with motor characteristics - 1DoF (account for dynamic variation in ua,up) ==
  volt : Inport  Port=1  LatchInput=off
  vel : Inport  Port=2  LatchInput=off
  Saturation1 : Saturate  UpperLimit=52.72  LowerLimit=-32.89
  axial flow dynamic : Subsystem  AncestorBlock=|
      | rov_design_analysis/Thruster
      | Modelling/Open-water propeller
      | characteristics/Thruster 1/T1
  "motor and propeller dynamic " : Subsystem  AncestorBlock=|
      | rov_design_analysis/Thruster
      | Modelling/Open-water propeller
      | characteristics/Thruster 1/Thrust 1
  Ta : Outport
  Qa : Outport  Port=2
  ua : Outport  Port=3
  wires:
  "motor and propeller dynamic "/2(Qa) -> Qa/1
  axial flow dynamic/1(ua) -> ua/1, "motor and propeller dynamic "/2(ua)
  vel/1 -> axial flow dynamic/2(vel)
  Saturation1/1 -> Ta/1, axial flow dynamic/1(Ta)
  "motor and propeller dynamic "/1(Ta) -> Saturation1/1
  volt/1 -> "motor and propeller dynamic "/1(volt)

== system rov_design_analysis/Propeller Models/2. propeller with motor characteristics - 1DoF (account for ua only) ==
  volt : Inport  Port=1  LatchInput=off
  Saturation1 : Saturate  UpperLimit=52.72  LowerLimit=-32.89
  "motor and propeller dynamic " : Subsystem  AncestorBlock=|
      | rov_design_analysis/Thruster
      | Modelling/Open-water propeller
      | characteristics/Thruster 1/Thrust 1
  Ta : Outport
  Qa : Outport  Port=2
  ua : Outport  Port=3
  wires:
  volt/1 -> "motor and propeller dynamic "/1(volt)
  "motor and propeller dynamic "/1(Ta) -> Saturation1/1
  Saturation1/1 -> Ta/1
  "motor and propeller dynamic "/2(Qa) -> Qa/1
  "motor and propeller dynamic "/3("ua ") -> "motor and propeller dynamic "/2(ua), ua/1

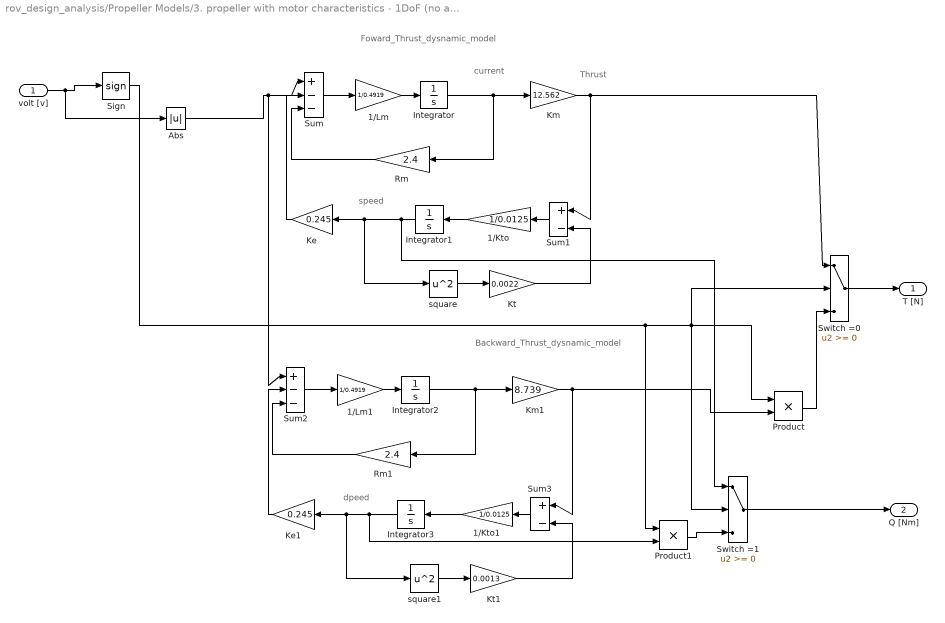
== system rov_design_analysis/Propeller Models/3. propeller with motor characteristics - 1DoF (no account for ua,up) ==
  note: Foward_Thrust_dysnamic_model
  note: Backward_Thrust_dysnamic_model
  note: Thrust
  note: current
  note: speed
  note: dpeed
  volt [v] : Inport  Port=1  LatchInput=off
  1/Kto : Gain  Orientation=left  Gain=1/0.0125  SaturateOnIntegerOverflow=on
  1/Kto1 : Gain  Orientation=left  Gain=1/0.0125  SaturateOnIntegerOverflow=on
  1/Lm : Gain  Gain=1/0.4919  SaturateOnIntegerOverflow=on
  1/Lm1 : Gain  Gain=1/0.4919  SaturateOnIntegerOverflow=on
  Abs : Abs  SaturateOnIntegerOverflow=on
  Integrator : Integrator
  Integrator1 : Integrator  Orientation=left
  Integrator2 : Integrator
  Integrator3 : Integrator  Orientation=left
  Ke : Gain  Orientation=left  Gain=0.245  SaturateOnIntegerOverflow=on
  Ke1 : Gain  Orientation=left  Gain=0.245  SaturateOnIntegerOverflow=on
  Km : Gain  Gain=12.562  SaturateOnIntegerOverflow=on
  Km1 : Gain  Gain=8.739  SaturateOnIntegerOverflow=on
  Kt : Gain  Gain=0.0022  SaturateOnIntegerOverflow=on
  Kt1 : Gain  Gain=0.0013  SaturateOnIntegerOverflow=on
  Product : Product  SaturateOnIntegerOverflow=on  RndMeth=Zero  InputSameDT=on
  Product1 : Product  SaturateOnIntegerOverflow=on  RndMeth=Zero  InputSameDT=on
  Rm : Gain  Orientation=left  Gain=2.4  SaturateOnIntegerOverflow=on
  Rm1 : Gain  Orientation=left  Gain=2.4  SaturateOnIntegerOverflow=on
  Sign : Signum
  Sum : Sum  Inputs=|+--  SaturateOnIntegerOverflow=on  InputSameDT=on
  Sum1 : Sum  Orientation=left  Inputs=|+-  SaturateOnIntegerOverflow=on  InputSameDT=on
  Sum2 : Sum  Inputs=|+--  SaturateOnIntegerOverflow=on  InputSameDT=on
  Sum3 : Sum  Orientation=left  Inputs=|+-  SaturateOnIntegerOverflow=on  InputSameDT=on
  Switch =0 : Switch  SaturateOnIntegerOverflow=on  InputSameDT=on
  Switch =1 : Switch  SaturateOnIntegerOverflow=on  InputSameDT=on
  square : Math  Operator=square  SaturateOnIntegerOverflow=on
  square1 : Math  Operator=square  SaturateOnIntegerOverflow=on
  T [N] : Outport
  Q [Nm] : Outport  Port=2
  wires:
  1/Lm1/1 -> Integrator2/1
  Rm1/1 -> Sum2/3
  Integrator2/1 -> Km1/1, Rm1/1
  1/Kto1/1 -> Integrator3/1
  Sum3/1 -> 1/Kto1/1
  Kt1/1 -> Sum3/2
  Integrator3/1 -> Ke1/1, square1/1, Product1/2
  Ke1/1 -> Sum2/2
  Sum2/1 -> 1/Lm1/1
  square1/1 -> Kt1/1
  1/Lm/1 -> Integrator/1
  Rm/1 -> Sum/3
  Sum/1 -> 1/Lm/1
  Integrator/1 -> Km/1, Rm/1
  1/Kto/1 -> Integrator1/1
  Sum1/1 -> 1/Kto/1
  Kt/1 -> Sum1/2
  Integrator1/1 -> Ke/1, square/1, Switch =1/1
  Ke/1 -> Sum/2
  square/1 -> Kt/1
  Km1/1 -> Sum3/1, Product/2
  Sign/1 -> Switch =0/2, Product/1, Switch =1/2, Product1/1
  Switch =0/1 -> T [N]/1
  Km/1 -> Sum1/1, Switch =0/1
  Product/1 -> Switch =0/3
  volt [v]/1 -> Sign/1, Abs/1
  Abs/1 -> Sum/1, Sum2/1
  Product1/1 -> Switch =1/3
  Switch =1/1 -> Q [Nm]/1

== system rov_design_analysis/Propeller Models/4. Open-water propeller characteristics ==
  n : Inport  Port=1  LatchInput=off
  Va : Inport  Port=2  LatchInput=off
  Dot Product1 : simulink/Math Operations/Dot Product  InputSameDT=on  OutDataType=sfix(16)  OutScaling=2^-10  DoSatur=off
  Dot Product2 : simulink/Math Operations/Dot Product  InputSameDT=on  OutDataType=sfix(16)  OutScaling=2^-10  DoSatur=off
  Kq poly : Constant  Value=Par_Thruster_Kqp
  Kt poly : Constant  Value=Par_Thruster_Ktp
  Math Function3 : Math  Operator=magnitude^2  SaturateOnIntegerOverflow=on
  Math Function4 : Math  Operator=magnitude^2  SaturateOnIntegerOverflow=on
  Mux1 : Mux  Inputs=3
  Product{2..3,6,9..10} (5 alike) : Product  SaturateOnIntegerOverflow=on
  Sign : Signum
  Switch : Switch  SaturateOnIntegerOverflow=on
  Zero limit : Saturate  UpperLimit=inf  LowerLimit=0
  Zero limit1 : Saturate  UpperLimit=inf  LowerLimit=0
  Zero limit2 : Saturate  UpperLimit=inf  LowerLimit=0
  reverse reduction : Gain  Gain=Par_Thruster_reverse_reduction  SaturateOnIntegerOverflow=on
  rhow[D^2 D^3 D^4] : Constant  Value=Glob_rhow*[Par_Thruster_D^2 Par_Thruster_D^3 Par_Thruster_D^4]
  "rhow[D^3 D^4 D^5] " : Constant  Value=Glob_rhow*[Par_Thruster_D^3 Par_Thruster_D^4 Par_Thruster_D^5]
  T_a : Outport
  Q_a : Outport  Port=2
  wires:
  Zero limit2/1 -> Product10/1, Math Function3/1
  Mux1/1 -> Dot Product1/2
  reverse reduction/1 -> Switch/3
  Switch/1 -> T_a/1
  Product2/1 -> reverse reduction/1, Switch/1
  Product3/1 -> Q_a/1
  Dot Product1/1 -> Zero limit/1
  Dot Product2/1 -> Zero limit1/1
  Zero limit/1 -> Product2/1
  Zero limit1/1 -> Product3/1
  Va/1 -> Zero limit2/1
  Sign/1 -> Product2/2, Switch/2, Product3/2
  Kt poly/1 -> Product6/1
  rhow[D^2 D^3 D^4]/1 -> Product6/2
  Product6/1 -> Dot Product1/1
  Kq poly/1 -> Product9/1
  "rhow[D^3 D^4 D^5] "/1 -> Product9/2
  Product9/1 -> Dot Product2/2
  n/1 -> Math Function4/1, Product10/2, Sign/1
  Math Function3/1 -> Mux1/1
  Math Function4/1 -> Mux1/3
  Product10/1 -> Mux1/2

== system rov_design_analysis/Propeller Models/5. first-order thruster dynamic - 4 DoF ==
  "volt " : Inport  Port=1  LatchInput=off
  Demux1 : Demux
  Mux2 : Mux
  SubSystem11 : Subsystem
  SubSystem12 : Subsystem
  SubSystem5 : Subsystem
  SubSystem6 : Subsystem
  "thrust " : Outport
  wires:
  "volt "/1 -> Demux1/1
  Mux2/1 -> "thrust "/1
  SubSystem11/1(thrust) -> Mux2/4
  Demux1/4 -> SubSystem11/1(volt)
  Demux1/3 -> SubSystem6/1(volt)
  SubSystem6/1(thrust) -> Mux2/3
  SubSystem5/1(thrust) -> Mux2/2
  Demux1/2 -> SubSystem5/1(volt)
  SubSystem12/1(thrust) -> Mux2/1
  Demux1/1 -> SubSystem12/1(volt)

== system rov_design_analysis/Propeller Models/6. first order motor dynamic- 1DoF (no account for ua,up) ==
  volt [v] : Inport  Port=1  LatchInput=off
  first order motor dynamic : Subsystem
  propeller Load Torque : Subsystem
  propeller thruster : Subsystem
  propeller Shaft Dynamic : Subsystem
  Ta : Outport
  Qa : Outport  Port=2
  wires:
  first order motor dynamic/1(torque) -> propeller Shaft Dynamic/1(Qm)
  propeller Shaft Dynamic/1(n) -> propeller Load Torque/1(n), propeller thruster/1(n)
  propeller Load Torque/1(Qa) -> Qa/1, propeller Shaft Dynamic/2(Qa)
  propeller thruster/1(Ta) -> Ta/1
  volt [v]/1 -> first order motor dynamic/1(volt)

== system rov_design_analysis/ROV Models/ Linear RRC ROV- unperturbed (6DoF) ==
  thrust : Inport  Port=1  LatchInput=off
  More Info : Subsystem  AncestorBlock=rov_design_analysis/ROV Models/Linear ROVRRC2 model/More Info
      settings: OpenFcn=|
      | clc
      | cd c:\Matlab7\toolbox\rov_design_analysis\\mat_file ;
      | load rrcrovf;
      mask Display: disp('Double-click here to load the\n linear RRCROV\n matrices')
  State-Space : StateSpace  A=At  B=Bt  C=Ct  D=Do
  vel : Outport
  wires:
  thrust/1 -> State-Space/1
  State-Space/1 -> vel/1

== system rov_design_analysis/ROV Models/ Pseudo Inverse (n X n-j), j<n ==
  In1 : Inport  Port=1  LatchInput=off
  Gain : Gain  Gain=pinv(T)  Multiplication=Matrix(K*u)
  Out1 : Outport
  wires:
  In1/1 -> Gain/1
  Gain/1 -> Out1/1
